simulink model "autoctlpre_hw_3"  (R2019a)
settings: Solver=VariableStepAuto  StartTime=0.0  StopTime=10.0  RelTol=1e-3
settings Model: Creator=70654  LastModifiedBy=70654

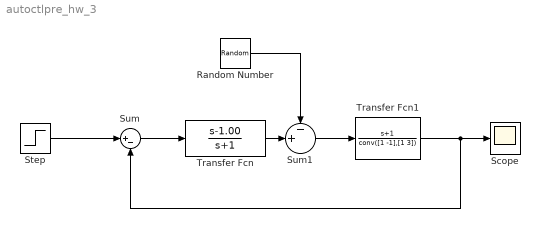
== system autoctlpre_hw_3 ==
  Random Number : RandomNumber  Variance=0  SampleTime=0.1
  Scope : Scope
  Step : Step  SampleTime=0
  Sum : Sum  Inputs=|+-
  Sum1 : Sum  Inputs=-+|
  Transfer Fcn : TransferFcn  Numerator=[1 -1.00]  Denominator=[1 1]
  Transfer Fcn1 : TransferFcn  Numerator=[1 1]  Denominator=conv([1 -1],[1 3])
  wires:
  Transfer Fcn1/1 -> Sum/2, Scope/1
  Sum/1 -> Transfer Fcn/1
  Step/1 -> Sum/1
  Random Number/1 -> Sum1/1
  Transfer Fcn/1 -> Sum1/2
  Sum1/1 -> Transfer Fcn1/1
